simulink model "simulink_design"  (R2019a)
settings: Solver=VariableStepAuto  StartTime=0.0  StopTime=10.0  RelTol=1e-3
values from neighbouring files (symbols this model uses):
  A = [0, 1, 0; 0, -b/J, k/J; 0, -k/L, -R/L]    [matlab.m]
  A_cl = [(A - B*K), (B*K); zeros(size(A)), (A - L*C)]    [matlab.m]
  B = [0; 0; 1/L]    [matlab.m]
  B_cl = [B; zeros(size(B))]    [matlab.m]
  C = [1, 0, 0]    [matlab.m]
  C_cl = [C, zeros(size(C))]    [matlab.m]
  D = 0    [matlab.m]
  D_cl = 0    [matlab.m]
  K = place(A, B, desired_controller_eigenvalues)    [matlab.m]
  L = place(A', C', desired_observer_eigenvalues)'    [matlab.m]
libraries: simulink x1
settings Model: Creator=AIMAL_KHAN  LastModifiedBy=AIMAL_KHAN

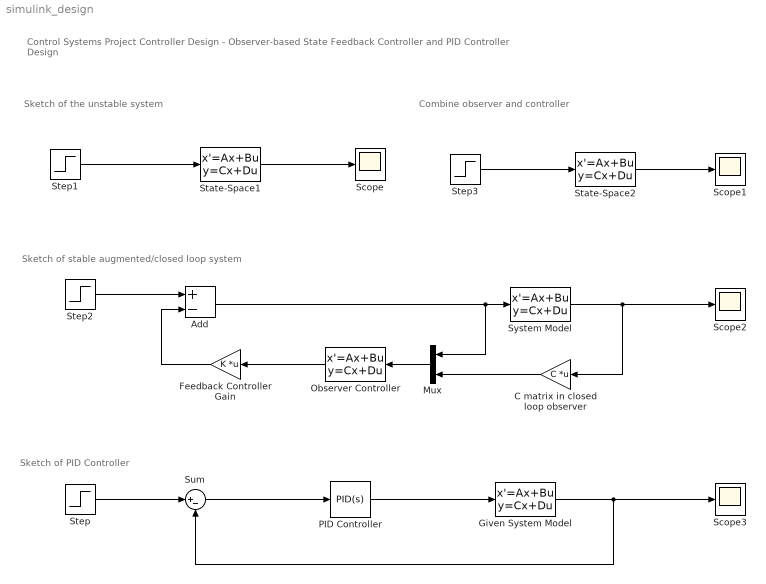
== system simulink_design ==
  note: Sketch of PID Controller
  note: Control Systems Project
      | Controller Design - Observer-based State Feedback Controller and PID Controller Design
  note: Combine observer and controller
  note: Sketch of stable augmented/closed loop system
  note: Sketch of the unstable system
  Add : Sum  Inputs=+-
  C matrix in closed loop observer : Gain  Gain=C  Multiplication=Matrix(K*u)
  Feedback Controller Gain : Gain  Gain=K  Multiplication=Matrix(K*u)
  Given System Model : StateSpace  A=A  B=B  C=C  D=D  InitialCondition=0
  Mux : Mux  Inputs=2
  Observer Controller : StateSpace  A=A-L*C  B=[B L]  C=eye(3)  D=[0 0; 0 0; 0 0]  InitialCondition=0
  PID Controller : simulink/Continuous/PID Controller  Controller=PID  Form=Parallel  TimeDomain=Continuous-time  SampleTime=-1  IntegratorMethod=Forward Euler  FilterMethod=Forward Euler  ControllerParametersSource=internal  P=646.656914598506  I=66.0541431240329  D=1025.12150339795  UseFilter=on  N=153.731998792333  TunerSelectOption=Transfer Function Based (PID Tuner App)  InitialConditionSource=internal  InitialConditionForIntegrator=0  InitialConditionForFilter=0  DifferentiatorICPrevScaledInput=0  ExternalReset=none  TrackingMode=off  Kt=1  LimitOutput=off  UpperSaturationLimit=inf  LowerSaturationLimit=-inf  LinearizeAsGain=on  AntiWindupMode=none  Kb=1  POutMin=[]  POutMax=[]  IOutMin=[]  IOutMax=[]  DOutMin=[]  DOutMax=[]  NOutMin=[]  NOutMax=[]  SumOutMin=[]  SumOutMax=[]  SaturationOutMin=[]  SaturationOutMax=[]  PParamMin=[]  PParamMax=[]  IParamMin=[]  IParamMax=[]  DParamMin=[]  DParamMax=[]  NParamMin=[]  NParamMax=[]  KbParamMin=[]  KbParamMax=[]  KtParamMin=[]  KtParamMax=[]  KbOutMin=[]  KbOutMax=[]  KtOutMin=[]  KtOutMax=[]  IntegratorOutMin=[]  IntegratorOutMax=[]  FilterOutMin=[]  FilterOutMax=[]  SumI1OutMin=[]  SumI1OutMax=[]  SumI2OutMin=[]  SumI2OutMax=[]  SumI3OutMin=[]  SumI3OutMax=[]  SumI4OutMin=[]  SumI4OutMax=[]  SumDOutMin=[]  SumDOutMax=[]  DifferentiatorOutMin=[]  DifferentiatorOutMax=[]  FilterDiffOutCoefMin=[]  FilterDiffOutCoefMax=[]  ReciprocalOutMin=[]  ReciprocalOutMax=[]  SumDenOutMin=[]  SumDenOutMax=[]  SumNumOutMin=[]  SumNumOutMax=[]  DivideOutMin=[]  DivideOutMax=[]  IntegratorContinuousStateAttributes=''  IntegratorStateMustResolveToSignalObject=off  IntegratorRTWStateStorageClass=Auto  FilterContinuousStateAttributes=''  FilterStateMustResolveToSignalObject=off  FilterRTWStateStorageClass=Auto  ParallelPVariant=InternalParameters  IdealPVariant=Disabled  IVariant=InternalParameters  DVariant=InternalParameters  IntegratorVariant=Continuous  SatVariant=Disabled  AWVariant=Passthrough  PCopyVariant=Disabled  TRVariant=Disabled  FdbkBlocksVariant=Forward  IdealPFdbkVariant=Disabled  SatFdbkVariant=Disabled  DerivativeFilterVariant=ContFilter  NVariant=InternalParameters  NCopyVariant=Disabled  FilterICVariant=InternalICsFilter  IntegratorICVariant=InternalICs  ExternalResetVariant=Disabled  TRSumVariant=Passthrough  SumFdbkVariant=Disabled  SumVariant=Sum_PID
  Scope{,1..3} (4 alike) : Scope
  State-Space1 : StateSpace  A=A  B=B  C=C  D=D  InitialCondition=0
  State-Space2 : StateSpace  A=A_cl  B=B_cl  C=C_cl  D=D_cl  InitialCondition=0
  Step{,1..3} (4 alike) : Step  SampleTime=0
  Sum : Sum  Inputs=|+-
  System Model : StateSpace  A=A  B=B  C=eye(3)  D=[0;0;0]  InitialCondition=0
  wires:
  Mux/1 -> Observer Controller/1
  Feedback Controller Gain/1 -> Add/2
  Add/1 -> Mux/1, System Model/1
  Step2/1 -> Add/1
  Observer Controller/1 -> Feedback Controller Gain/1
  State-Space2/1 -> Scope1/1
  Step3/1 -> State-Space2/1
  Step1/1 -> State-Space1/1
  C matrix in closed loop observer/1 -> Mux/2
  System Model/1 -> C matrix in closed loop observer/1, Scope2/1
  State-Space1/1 -> Scope/1
  Step/1 -> Sum/1
  Sum/1 -> PID Controller/1
  PID Controller/1 -> Given System Model/1
  Given System Model/1 -> Scope3/1, Sum/2
